simulink model "Lab3_P4_AB"  (R2020b)
settings: Solver=VariableStepAuto  StartTime=0.0  StopTime=20  MaxStep=2e-2  RelTol=1e-3
libraries: simulink x1
settings Model: Creator=rodsc  LastModifiedBy=rodsc
settings SolverCC: ZeroCrossAlgorithm=Adaptive
settings DebuggingCC: IgnoredZcDiagnostic=none
settings SFSimCC: SimCustomSourceCode=parede.c  SimCustomHeaderCode="#include \"parede.h\""  SimUserSources=parede.c  SimParseCustomCode=off

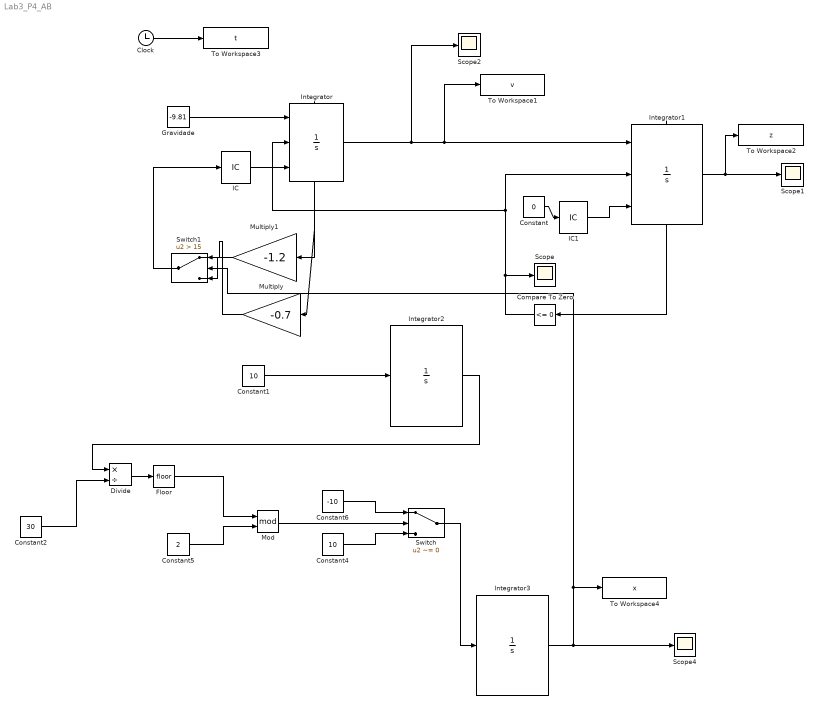
== system Lab3_P4_AB ==
  Clock : Clock
  Compare To Zero : simulink/Logic and Bit Operations/Compare To Zero  relop=<=  OutDataTypeStr=boolean
  Constant : Constant  Value=0
  Constant1 : Constant  Value=10
  Constant2 : Constant  Value=30
  Constant4 : Constant  Value=10
  Constant5 : Constant  Value=2
  Constant6 : Constant  Value=-10
  Divide : Product  Inputs=*/
  Floor : Rounding
  "Gravidade " : Constant  Value=-9.81
  IC : InitialCondition  Value=0
  IC1 : InitialCondition  Value=10
  Integrator : Integrator  ExternalReset=rising  InitialConditionSource=external  ShowStatePort=on
  Integrator1 : Integrator  ExternalReset=rising  InitialConditionSource=external  LimitOutput=on  LowerSaturationLimit=0  ShowStatePort=on
  Integrator2 : Integrator  LowerSaturationLimit=0
  Integrator3 : Integrator  LimitOutput=on  LowerSaturationLimit=0
  Mod : Math  Operator=mod  SaturateOnIntegerOverflow=on
  Multiply : Gain  Gain=-0.7
  Multiply1 : Gain  Gain=-1.2
  Scope{,1..2,4} (4 alike) : Scope
  Switch : Switch  Criteria=u2 ~= 0
  Switch1 : Switch  Criteria=u2 > Threshold  Threshold=15
  To Workspace1 : ToWorkspace  VariableName=v  SampleTime=-1
      settings: Save2DSignal=2-D array (concatenate along first dimension)
  To Workspace2 : ToWorkspace  VariableName=z  SampleTime=-1
      settings: Save2DSignal=2-D array (concatenate along first dimension)
  To Workspace3 : ToWorkspace  VariableName=t  SampleTime=-1
      settings: Save2DSignal=2-D array (concatenate along first dimension)
  To Workspace4 : ToWorkspace  VariableName=x  SampleTime=-1
      settings: Save2DSignal=2-D array (concatenate along first dimension)
  wires:
  "Gravidade "/1 -> Integrator/1
  IC/1 -> Integrator/3
  Integrator/1 -> Scope2/1, To Workspace1/1, Integrator1/1
  Integrator1/State -> Compare To Zero/1
  Compare To Zero/1 -> Integrator/2, Integrator1/2, Scope/1
  Constant/1 -> IC1/1
  IC1/1 -> Integrator1/3
  Integrator1/1 -> To Workspace2/1, Scope1/1
  Clock/1 -> To Workspace3/1
  Integrator2/1 -> Divide/1
  Integrator/State -> Multiply/1, Multiply1/1
  Constant1/1 -> Integrator2/1
  Floor/1 -> Mod/1
  Divide/1 -> Floor/1
  Constant2/1 -> Divide/2
  Constant5/1 -> Mod/2
  Integrator3/1 -> Switch1/2, To Workspace4/1, Scope4/1
  Mod/1 -> Switch/2
  Constant4/1 -> Switch/3
  Constant6/1 -> Switch/1
  Switch/1 -> Integrator3/1
  Switch1/1 -> IC/1
  Multiply1/1 -> Switch1/3
  Multiply/1 -> Switch1/1
